simulink model "Car_14DOF_Lat_Long_Control_FINAL"  (R2024b)
settings: Solver=ode4  StartTime=0.0  StopTime=60  FixedStep=0.001  RelTol=1e-3
undefined symbols (not defined in the file): Ar1, Ar2, Ar3, Ar4, b, c, C_alpha, C_line, C_sigma, curvature, f, g, gradbp, Iw, Ix, Iy, Iz, k, ki, kp, kR, Kz1, Kz2, Kz3, L, L1, L2, lf, lh, lh_vis, lr, lw, m, mR, psi0, reff, uFz, Vx_ref, wc, x0, xRef2s, y0, yRef2s, z0
libraries: vehdynlibviscommon x1, deeplib x1
settings Model: Creator=sherlock2204  LastModifiedBy=sherlock2204
settings DebuggingCC: SigSpecEnsureSampleTimeMsg=none

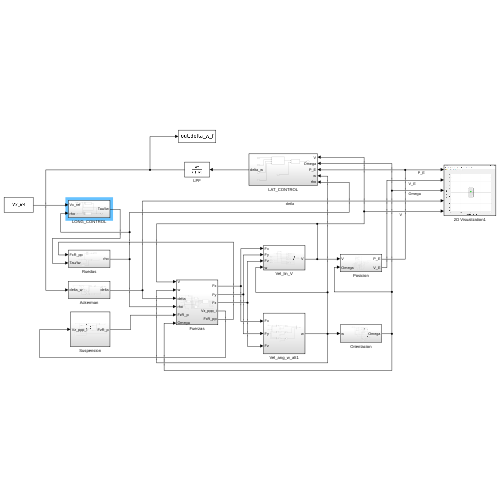
[thumbnail: Simulink's stored preview of the top-level diagram]
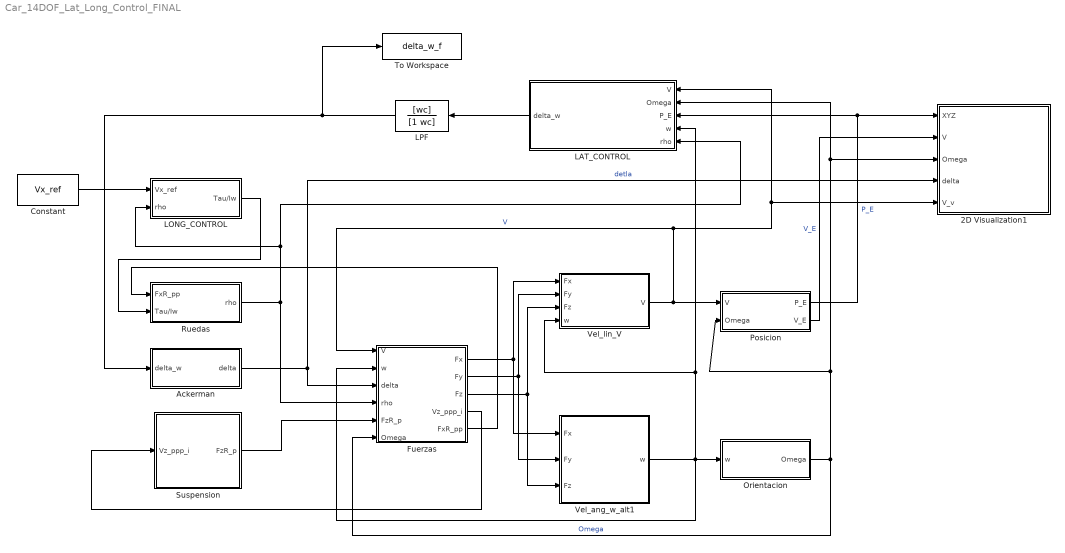
== system Car_14DOF_Lat_Long_Control_FINAL ==
  2D Visualization1 : Subsystem
      mask Display: image("visualization.JPG");
  Ackerman : Subsystem
  Constant : Constant  Value=Vx_ref
  Fuerzas : Subsystem
  LAT_CONTROL : Subsystem
  LONG_CONTROL : Subsystem
  LPF : TransferFcn  Numerator=[wc]  Denominator=[1 wc]
  Orientacion : Subsystem
  Posicion : Subsystem
  Ruedas : Subsystem
  Suspension : Subsystem
  To Workspace : ToWorkspace  VariableName=delta_w_f  SaveFormat=Timeseries  SampleTime=-1
  Vel_ang_w_alt1 : Subsystem
  Vel_lin_V : Subsystem
  wires:
  Fuerzas/3(Fz) -> Vel_ang_w_alt1/3(Fz), Vel_lin_V/3(Fz)
  Vel_ang_w_alt1/1(w) -> Vel_lin_V/4(w), LAT_CONTROL/4(w), Orientacion/1(w), Fuerzas/2(w)
  Vel_lin_V/1(V) -> Fuerzas/1(V), LAT_CONTROL/1(V), 2D Visualization1/5(V_v), Posicion/1(V)  "V"
  Suspension/1(FzR_p) -> Fuerzas/5(FzR_p)
  Fuerzas/4(Vz_ppp_i) -> Suspension/1(Vz_ppp_i)
  Ackerman/1(delta) -> Fuerzas/3(delta), 2D Visualization1/4(delta)  "detla"
  Fuerzas/1(Fx) -> Vel_ang_w_alt1/1(Fx), Vel_lin_V/1(Fx)
  Fuerzas/2(Fy) -> Vel_ang_w_alt1/2(Fy), Vel_lin_V/2(Fy)
  Orientacion/1(Omega) -> LAT_CONTROL/2(Omega), 2D Visualization1/3(Omega), Posicion/2(Omega), Fuerzas/6(Omega)  "Omega"
  Posicion/2(V_E) -> 2D Visualization1/2(V)  "V_E"
  Posicion/1(P_E) -> 2D Visualization1/1(XYZ), LAT_CONTROL/3(P_E)  "P_E"
  Fuerzas/5(FxR_pp) -> Ruedas/1(FxR_pp)
  Ruedas/1(rho) -> Fuerzas/4(rho), LAT_CONTROL/5(rho), LONG_CONTROL/2(rho)
  Constant/1 -> LONG_CONTROL/1(Vx_ref)
  LONG_CONTROL/1(Tau/Iw) -> Ruedas/2(Tau/Iw)
  LPF/1 -> To Workspace/1, Ackerman/1(delta_w)
  LAT_CONTROL/1(delta_w) -> LPF/1

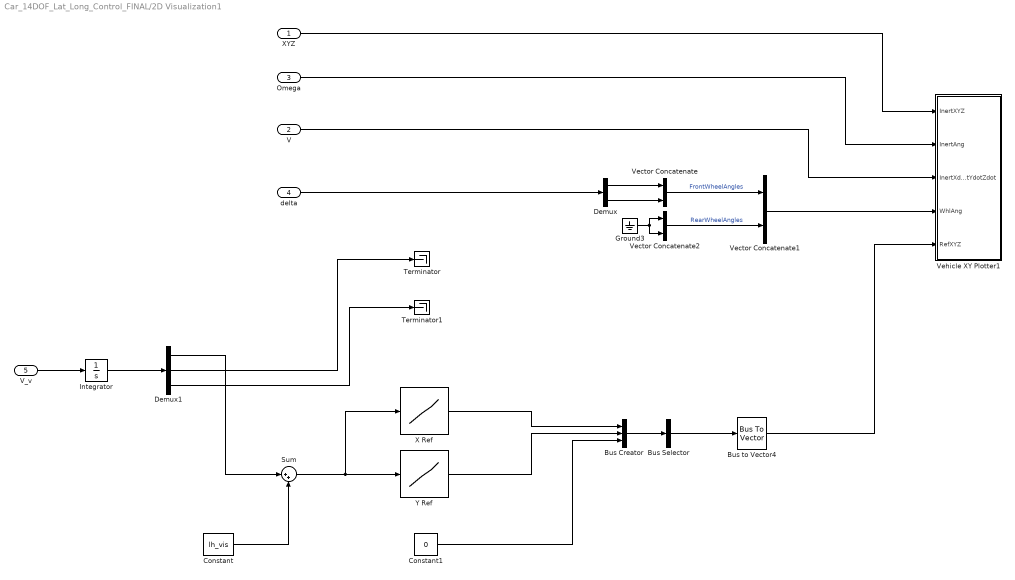
== system Car_14DOF_Lat_Long_Control_FINAL/2D Visualization1 ==
  XYZ : Inport
  V : Inport  Port=2
  Omega : Inport  Port=3
  delta : Inport  Port=4
  V_v : Inport  Port=5
  Bus Creator : BusCreator  Inputs=3
  Bus Selector : BusSelector  OutputSignals=signal1,signal2,signal3  OutputAsBus=on
  Bus to Vector4 : BusToVector
  Constant : Constant  Value=lh_vis
  Constant1 : Constant  Value=0
  Demux : Demux  Outputs=2
  Demux1 : Demux  Outputs=3
  Ground3 : Ground
  Integrator : Integrator
  Sum : Sum  Inputs=|++
  Terminator : Terminator
  Terminator1 : Terminator
  Vector Concatenate : Concatenate
  Vector Concatenate1 : Concatenate
  Vector Concatenate2 : Concatenate
  Vehicle XY Plotter1 : Subsystem  mask(Vehicle XY Plotter){extRef=on, extStats=off, extTireF=off, a=lf, b=lr, w=c, figBorder=10, bufferSize=1024, velNorm=5, tireFNorm=1000, pltDT=0.2}
      mask prompts: extRef "Plot path reference, extRef"; extStats "Display speed, RPM and Gear"; extTireF "Display tire forces"; a "Distance to front axle from CG, a [m]:"; b "Distance to rear axle from CG, b [m]:"; w "Track width, w [m]:"; figBorder "Distance to figure borders, figBorder [m]:"; bufferSize "Path buffer sampe size, bufferSize []:"; velNorm "Velocity vector scaling, velNorm [m*s/m]:"; tireFNorm "Tire force vector scaling, tireFNorm [m/N]:"; pltDT "Plot update rate, pltDT [s]:"
      mask help:
      | This block will display a MATLAB figure which indicates the vehicle path, current position and heading velocity.
      | An optional path reference is also provided.
      mask init:
      | block = gcb;
      | if autoblkschecksimstopped(block)
      |     ParamNames = {'extRef';'extStats';'extTireF';'extTireF'};
      |     PortNames = {'RefXYZ';'Stats';'TireFx';'TireFy'};
      |     for idx=1:length(PortNames)
      |         InportOption  = {'built-in/Ground', [PortNames{idx}, ' Ground'];...
      |             'built-in/Inport',PortNames{idx}};
      |         if ~strcmp(get_param(block,ParamNames{idx}),'on')
      |             NewBlkHdl = autoblksreplaceblock(block, InportOption, 1);
      |             set_param(NewBlkHdl, 'ShowName', 'off');
      |         else
      |             autoblksreplaceblock(block, InportOption, 2);
      |         end
      |     end
      |     InportNames = {'InertXYZ';'InertAng';'InertXdotYdotZdot';'WhlAng';'RefXYZ';'Stats';'TireFx';'TireFy'};
      |     FoundNames = get_param(find_system(block, 'LookUnderMasks', 'all', 'SearchDepth', 1, 'FollowLinks', 'on', 'BlockType', 'Inport'), 'Name');
      |     [~,PortI] = intersect(InportNames, FoundNames);
      |     PortI = sort(PortI);
      |     for idx = 1:length(PortI)
      |         set_param([block, '/', InportNames{PortI(idx)}], 'Port', num2str(idx));
      |     end
      | end
      mask TypeOptions a: Vehicle XY Plotter/a
      mask TypeOptions b: Vehicle XY Plotter/b
      mask TypeOptions w: Vehicle XY Plotter/w
      mask TypeOptions figBorder: Vehicle XY Plotter/figBorder
      mask TypeOptions bufferSize: Vehicle XY Plotter/bufferSize
      mask TypeOptions velNorm: Vehicle XY Plotter/velNorm
      mask TypeOptions tireFNorm: Vehicle XY Plotter/tireFNorm
      mask DialogControl Container3 Prompt: Plot and Display Options
  X Ref : Lookup_n-D  NumberOfTableDimensions=1  BreakpointsForDimension1=gradbp  Table=xRef2s  InternalRulePriority=Speed  RndMeth=Simplest
  Y Ref : Lookup_n-D  NumberOfTableDimensions=1  BreakpointsForDimension1=gradbp  Table=yRef2s  InternalRulePriority=Speed  RndMeth=Simplest
  wires:
  Omega/1 -> Vehicle XY Plotter1/2(InertAng)
  XYZ/1 -> Vehicle XY Plotter1/1(InertXYZ)
  V/1 -> Vehicle XY Plotter1/3(InertXdotYdotZdot)
  Vector Concatenate2/1 -> Vector Concatenate1/2  "RearWheelAngles"
  Vector Concatenate/1 -> Vector Concatenate1/1  "FrontWheelAngles"
  Ground3/1 -> Vector Concatenate2/2, Vector Concatenate2/1
  Vector Concatenate1/1 -> Vehicle XY Plotter1/4(WhlAng)
  delta/1 -> Demux/1
  Demux/1 -> Vector Concatenate/1
  Demux/2 -> Vector Concatenate/2
  Bus Creator/1 -> Bus Selector/1
  Y Ref/1 -> Bus Creator/2
  Bus Selector/1 -> Bus to Vector4/1
  Demux1/3 -> Terminator1/1
  X Ref/1 -> Bus Creator/1
  Constant1/1 -> Bus Creator/3
  Bus to Vector4/1 -> Vehicle XY Plotter1/5(RefXYZ)
  Demux1/2 -> Terminator/1
  V_v/1 -> Integrator/1
  Integrator/1 -> Demux1/1
  Demux1/1 -> Sum/1
  Sum/1 -> X Ref/1, Y Ref/1
  Constant/1 -> Sum/2

== system Car_14DOF_Lat_Long_Control_FINAL/Ackerman ==
  delta_w : Inport
  Atan : Trigonometry  Operator=atan
  Atan1 : Trigonometry  Operator=atan
  Constant : Constant  Value=L
  Divide : Product  Inputs=*/
  Divide1 : Product  Inputs=*/
  Gain : Gain  Gain=L
  Gain1 : Gain  Gain=lw
  Mux : Mux  Inputs=2
  Sum : Sum  Inputs=++|
  Sum1 : Sum  Inputs=-+|
  Tan : Trigonometry  Operator=tan
  delta : Outport
  wires:
  Mux/1 -> delta/1
  delta_w/1 -> Tan/1
  Tan/1 -> Gain/1, Gain1/1
  Gain/1 -> Divide1/1, Divide/1
  Divide/1 -> Atan/1
  Constant/1 -> Sum/2, Sum1/2
  Gain1/1 -> Sum/1, Sum1/1
  Sum/1 -> Divide/2
  Sum1/1 -> Divide1/2
  Divide1/1 -> Atan1/1
  Atan/1 -> Mux/1
  Atan1/1 -> Mux/2

== system Car_14DOF_Lat_Long_Control_FINAL/Fuerzas ==
  V : Inport
  w : Inport  Port=2
  delta : Inport  Port=3
  rho : Inport  Port=4
  FzR_p : Inport  Port=5
  Omega : Inport  Port=6
  Demux : Demux  Outputs=2
  Demux1 : Demux  Outputs=3
  M_Fuerzas : Subsystem
  Terminator : Terminator
  Vel_transf : Subsystem
  alpha_alt3 : Subsystem
  sigma_alt0 : Subsystem
  Fx : Outport
  Fy : Outport  Port=2
  Fz : Outport  Port=3
  Vz_ppp_i : Outport  Port=4
  FxR_pp : Outport  Port=5
  wires:
  V/1 -> Vel_transf/1(V)
  w/1 -> Vel_transf/2(w)
  Demux1/1 -> Vel_transf/3(phi), M_Fuerzas/5(phi)  "phi"
  Demux1/2 -> M_Fuerzas/6(theta), Vel_transf/4(theta)  "theta"
  M_Fuerzas/2(Fy) -> Fy/1
  M_Fuerzas/3(Fz) -> Fz/1
  delta/1 -> Vel_transf/5(delta), Demux/1
  Demux/2 -> alpha_alt3/4(delta_3), M_Fuerzas/4(delta_3)
  Demux/1 -> M_Fuerzas/3(delta_1), alpha_alt3/3(delta_1)
  rho/1 -> sigma_alt0/2(rho)
  Vel_transf/1(Vx_ppp_i) -> sigma_alt0/1(Vx_ppp_i)
  sigma_alt0/1(sigma) -> M_Fuerzas/1(sigma)
  alpha_alt3/1(alpha) -> M_Fuerzas/2(alpha)
  FzR_p/1 -> M_Fuerzas/7(FzR_p)
  Vel_transf/2(Vz_ppp_i) -> Vz_ppp_i/1
  Vel_transf/3(Vx_pp_i) -> alpha_alt3/1(Vx_pp_i)
  Vel_transf/4(Vy_pp_i) -> alpha_alt3/2(Vy_pp_i)
  Omega/1 -> Demux1/1
  Demux1/3 -> Terminator/1  "psi"
  M_Fuerzas/4(FxR_pp) -> FxR_pp/1
  M_Fuerzas/1(Fx) -> Fx/1

== system Car_14DOF_Lat_Long_Control_FINAL/LAT_CONTROL ==
  V : Inport
  Omega : Inport  Port=2
  P_E : Inport  Port=3
  w : Inport  Port=4
  rho : Inport  Port=5
  BACK_STEPPING_1 : Subsystem
  LSTM_NETWORK : Subsystem
  delta_w : Outport
  wires:
  V/1 -> BACK_STEPPING_1/1(V)
  Omega/1 -> BACK_STEPPING_1/2(Omega)
  P_E/1 -> BACK_STEPPING_1/3(P_E)
  w/1 -> BACK_STEPPING_1/4(w)
  rho/1 -> LSTM_NETWORK/2(rho)
  LSTM_NETWORK/1(delta_w) -> delta_w/1
  BACK_STEPPING_1/1(Tau_z) -> LSTM_NETWORK/1(Tau_z)

== system Car_14DOF_Lat_Long_Control_FINAL/LONG_CONTROL ==
  Vx_ref : Inport
  rho : Inport  Port=2
  ADRC : Subsystem
  ESO : Subsystem
  Tau/Iw : Outport
  wires:
  rho/1 -> ESO/1(x1), ADRC/1(x1)
  ADRC/1(u) -> Tau/Iw/1, ESO/2(u)  "u=Tau/Iw"
  ESO/1(hat_x2) -> ADRC/3(hat_x2)
  Vx_ref/1 -> ADRC/2(x1_ref)

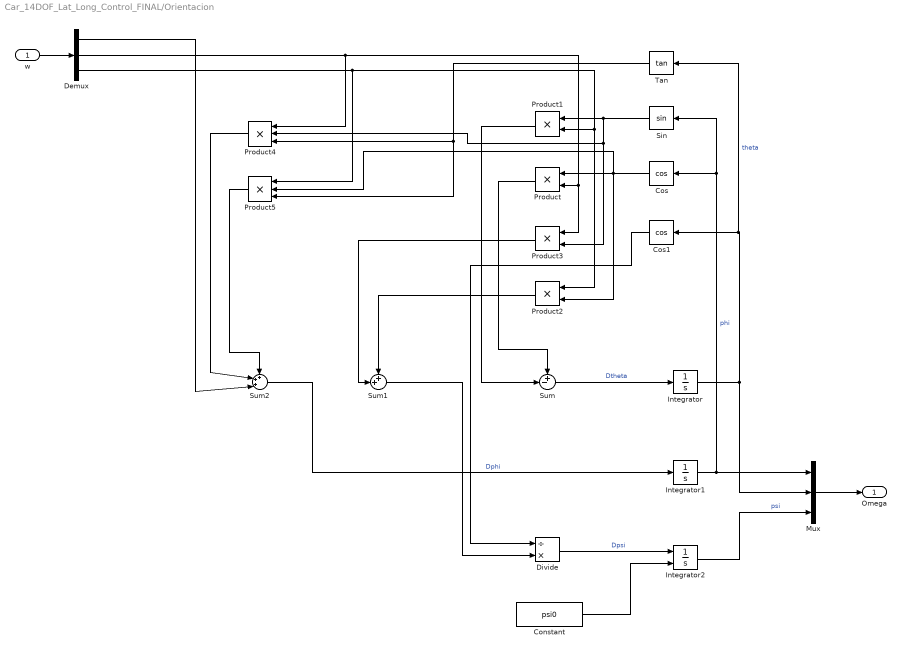
== system Car_14DOF_Lat_Long_Control_FINAL/Orientacion ==
  w : Inport
  Constant : Constant  Value=psi0
  Cos : Trigonometry  Operator=cos
  Cos1 : Trigonometry  Operator=cos
  Demux : Demux  Outputs=3
  Divide : Product  Inputs=/*
  Integrator : Integrator
  Integrator1 : Integrator
  Integrator2 : Integrator  InitialConditionSource=external
  Mux : Mux  Inputs=3
  Product{,1..3} (4 alike) : Product
  Product4 : Product  Inputs=3
  Product5 : Product  Inputs=3
  Sin : Trigonometry
  Sum : Sum  Inputs=+-|
  Sum1 : Sum  Inputs=++|
  Sum2 : Sum  Inputs=+++|
  Tan : Trigonometry  Operator=tan
  Omega : Outport
  wires:
  w/1 -> Demux/1
  Integrator/1 -> Mux/2, Tan/1, Cos1/1  "theta"
  Integrator2/1 -> Mux/3  "psi"
  Sin/1 -> Product4/2, Product3/2, Product1/1
  Cos/1 -> Product5/2, Product2/2, Product/1
  Demux/2 -> Product4/1, Product3/1, Product/2
  Demux/3 -> Product5/1, Product2/1, Product1/2
  Product/1 -> Sum/1
  Product1/1 -> Sum/2
  Sum/1 -> Integrator/1  "Dtheta"
  Integrator1/1 -> Sin/1, Cos/1, Mux/1  "phi"
  Product2/1 -> Sum1/1
  Product3/1 -> Sum1/2
  Divide/1 -> Integrator2/1  "Dpsi"
  Sum1/1 -> Divide/2
  Cos1/1 -> Divide/1
  Tan/1 -> Product4/3, Product5/3
  Sum2/1 -> Integrator1/1  "Dphi"
  Product5/1 -> Sum2/1
  Product4/1 -> Sum2/2
  Demux/1 -> Sum2/3
  Mux/1 -> Omega/1
  Constant/1 -> Integrator2/2

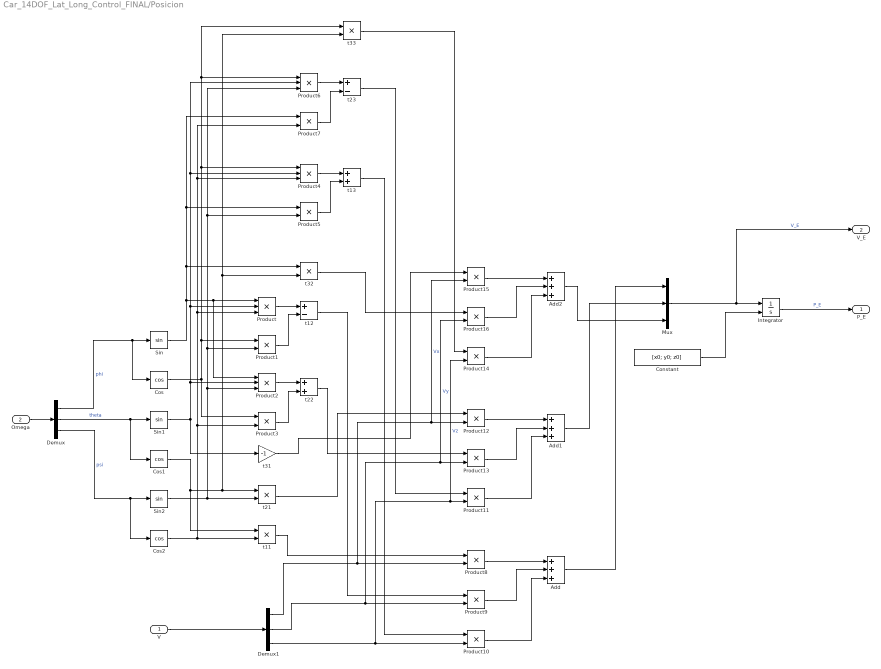
== system Car_14DOF_Lat_Long_Control_FINAL/Posicion ==
  V : Inport
  Omega : Inport  Port=2
  Add : Sum  Inputs=+++
  Add1 : Sum  Inputs=+++
  Add2 : Sum  Inputs=+++
  Constant : Constant  Value=[x0; y0; z0]
  Cos : Trigonometry  Operator=cos
  Cos1 : Trigonometry  Operator=cos
  Cos2 : Trigonometry  Operator=cos
  Demux : Demux  Outputs=3
  Demux1 : Demux  Outputs=3
  Integrator : Integrator  InitialConditionSource=external
  Mux : Mux  Inputs=3
  Product{,2,4,6} (4 alike) : Product  Inputs=3
  Product{1,3,5,7..16} (13 alike) : Product
  Sin : Trigonometry
  Sin1 : Trigonometry
  Sin2 : Trigonometry
  t{11,21,32..33} (4 alike) : Product
  t12 : Sum  Inputs=+-
  t13 : Sum
  t22 : Sum
  t23 : Sum  Inputs=+-
  t31 : Gain  Gain=-1
  P_E : Outport
  V_E : Outport  Port=2
  wires:
  Demux/1 -> Cos/1, Sin/1  "phi"
  Demux/2 -> Cos1/1, Sin1/1  "theta"
  Demux/3 -> Cos2/1, Sin2/1  "psi"
  Omega/1 -> Demux/1
  Cos2/1 -> Product7/2, Product4/3, Product/3, Product3/2, t11/2
  Cos1/1 -> t21/1, t33/2, t32/2, t11/1
  Sin2/1 -> Product6/3, Product5/2, Product1/2, Product2/3, t21/2
  Sin1/1 -> Product6/2, Product4/2, Product/2, Product2/2, t31/1
  Sin/1 -> Product7/1, Product5/1, t32/1, Product2/1, Product/1
  Cos/1 -> t33/1, Product6/1, Product4/1, Product1/1, Product3/1
  Product/1 -> t12/1
  Product1/1 -> t12/2
  Product3/1 -> t22/2
  Product2/1 -> t22/1
  Product5/1 -> t13/2
  Product4/1 -> t13/1
  Product6/1 -> t23/1
  Product7/1 -> t23/2
  V/1 -> Demux1/1
  Demux1/1 -> Product15/2, Product12/2, Product8/2  "Vx"
  Demux1/3 -> Product10/2, Product14/2, Product11/2  "Vz"
  Demux1/2 -> Product9/2, Product16/2, Product13/2  "Vy"
  t11/1 -> Product8/1
  t12/1 -> Product9/1
  t13/1 -> Product10/1
  Product8/1 -> Add/1
  Product9/1 -> Add/2
  Product10/1 -> Add/3
  Product13/1 -> Add1/2
  Product12/1 -> Add1/1
  Product11/1 -> Add1/3
  t21/1 -> Product12/1
  t22/1 -> Product13/1
  t23/1 -> Product11/1
  Product15/1 -> Add2/1
  Product16/1 -> Add2/2
  Product14/1 -> Add2/3
  t31/1 -> Product15/1
  t32/1 -> Product16/1
  t33/1 -> Product14/1
  Add/1 -> Mux/1
  Add1/1 -> Mux/2
  Add2/1 -> Mux/3
  Mux/1 -> V_E/1, Integrator/1  "V_E"
  Integrator/1 -> P_E/1  "P_E"
  Constant/1 -> Integrator/2

== system Car_14DOF_Lat_Long_Control_FINAL/Ruedas ==
  FxR_pp : Inport
  Tau/Iw : Inport  Port=2
  Add1 : Sum  Inputs=++++
  Constant : Constant  Value=0.0001*[1 1 1 1]
  Demux : Demux
  Gain : Gain
  Gain13 : Gain  Gain=reff/Iw
  Gain3 : Gain  Gain=1/4
  Integrator4 : Integrator  InitialConditionSource=external
  Sum : Sum  Inputs=|+-
  To Workspace : ToWorkspace  VariableName=tau_w  SaveFormat=Timeseries  SampleTime=-1
  rho : Outport
  wires:
  FxR_pp/1 -> Gain13/1
  Tau/Iw/1 -> Gain/1  "u=Tau/Iw"
  Sum/1 -> Integrator4/1  "Drho"
  Gain13/1 -> Sum/2  "EPS(t)"
  Gain/1 -> Demux/1, Sum/1  "Tau"
  Integrator4/1 -> rho/1
  Constant/1 -> Integrator4/2
  Add1/1 -> Gain3/1
  Demux/3 -> Add1/3
  Demux/2 -> Add1/2
  Demux/1 -> Add1/1
  Demux/4 -> Add1/4
  Gain3/1 -> To Workspace/1

== system Car_14DOF_Lat_Long_Control_FINAL/Suspension ==
  Vz_ppp_i : Inport
  Add : Sum  Inputs=--
  Add1 : Sum  Inputs=++-
  Constant2 : Constant  Value=[0;0;0;0]
  Constant3 : Constant  Value=[0;0;0;0]
  Constant4 : Constant  Value=[0;0;0;0]
  Gain : Gain  Gain=b
  Gain1 : Gain  Gain=k
  Gain4 : Gain  Gain=1/mR
  Gain7 : Gain  Gain=kR
  Integrator2 : Integrator  InitialConditionSource=external
  Integrator3 : Integrator  InitialConditionSource=external
  Integrator4 : Integrator  InitialConditionSource=external
  Sum : Sum  Inputs=|+-
  Sum2 : Sum  Inputs=|+-
  FzR_p : Outport
  wires:
  Sum/1 -> Gain/1
  Integrator3/1 -> Gain7/1, Sum2/2  "zR"
  Sum2/1 -> Gain1/1
  Add/1 -> FzR_p/1
  Add1/1 -> Gain4/1
  Gain/1 -> Add1/1, Add/1
  Integrator2/1 -> Integrator3/1, Sum/2  "DzR"
  Gain1/1 -> Add1/2, Add/2
  Gain4/1 -> Integrator2/1
  Constant4/1 -> Integrator2/2
  Constant3/1 -> Integrator3/2
  Vz_ppp_i/1 -> Integrator4/1, Sum/1  "DzA"
  Integrator4/1 -> Sum2/1  "zA"
  Constant2/1 -> Integrator4/2
  Gain7/1 -> Add1/3

== system Car_14DOF_Lat_Long_Control_FINAL/Vel_ang_w_alt1 ==
  Fx : Inport
  Fy : Inport  Port=2
  Fz : Inport  Port=3
  Integrator : Integrator  InitialConditionSource=external
  Integrator1 : Integrator  InitialConditionSource=external
  Integrator2 : Integrator  InitialConditionSource=external
  Multiply : Gain  Gain=(1/Ix)*[c c -c -c lh lh lh lh]  Multiplication=Matrix(K*u) (u vector)
  Multiply1 : Gain  Gain=(1/Iy)*[-lh -lh -lh -lh -lf lr -lf lr]  Multiplication=Matrix(K*u) (u vector)
  Multiply2 : Gain  Gain=(1/Iz)*[lf -lr lf -lr -c -c c c]  Multiplication=Matrix(K*u) (u vector)
  Mux : Mux  Inputs=3
  Vector Concatenate : Concatenate
  Vector Concatenate1 : Concatenate
  Vector Concatenate2 : Concatenate
  wx0 : Constant  Value=0
  wy0 : Constant  Value=0
  wz0 : Constant  Value=0
  w : Outport
  wires:
  wx0/1 -> Integrator/2
  wy0/1 -> Integrator1/2
  Mux/1 -> w/1
  wz0/1 -> Integrator2/2
  Integrator/1 -> Mux/1  "wx"
  Fz/1 -> Vector Concatenate/1, Vector Concatenate1/2
  Fy/1 -> Vector Concatenate/2, Vector Concatenate2/1
  Vector Concatenate/1 -> Multiply/1
  Multiply1/1 -> Integrator1/1
  Vector Concatenate1/1 -> Multiply1/1
  Fx/1 -> Vector Concatenate2/2, Vector Concatenate1/1
  Integrator1/1 -> Mux/2  "wy"
  Vector Concatenate2/1 -> Multiply2/1
  Integrator2/1 -> Mux/3  "wz"
  Multiply/1 -> Integrator/1
  Multiply2/1 -> Integrator2/1

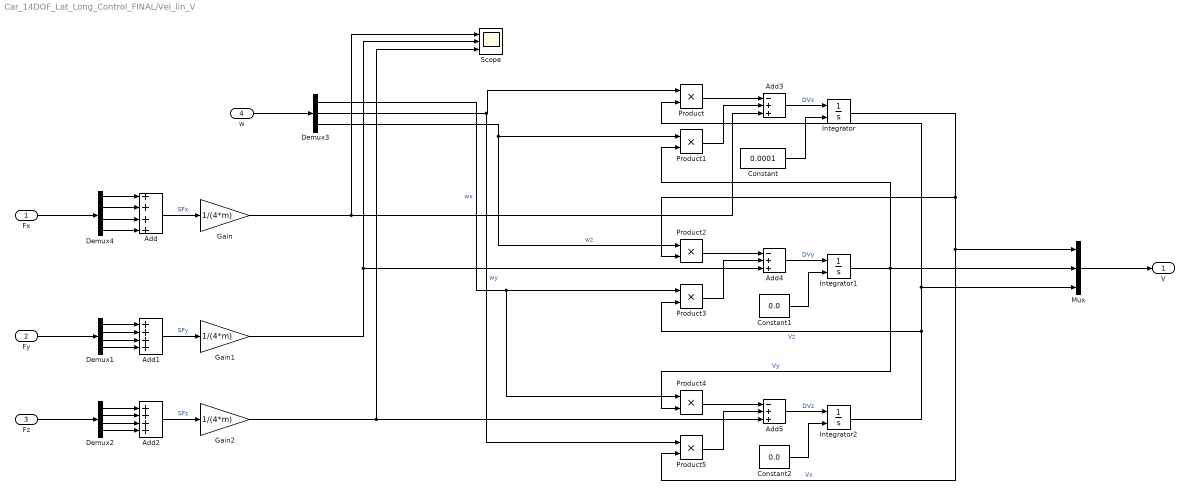
== system Car_14DOF_Lat_Long_Control_FINAL/Vel_lin_V ==
  Fx : Inport
  Fy : Inport  Port=2
  Fz : Inport  Port=3
  w : Inport  Port=4
  Add : Sum  Inputs=++++
  Add1 : Sum  Inputs=++++
  Add2 : Sum  Inputs=++++
  Add3 : Sum  Inputs=-++
  Add4 : Sum  Inputs=-++
  Add5 : Sum  Inputs=-++
  Constant : Constant  Value=0.0001  SampleTime=0.001
  Constant1 : Constant  Value=0.0
  Constant2 : Constant  Value=0.0
  Demux1 : Demux
  Demux2 : Demux
  Demux3 : Demux  Outputs=3
  Demux4 : Demux
  Gain : Gain  Gain=1/(4*m)
  Gain1 : Gain  Gain=1/(4*m)
  Gain2 : Gain  Gain=1/(4*m)
  Integrator : Integrator  InitialConditionSource=external  UpperSaturationLimit=27.7778  LowerSaturationLimit=-27.7778  AbsoluteTolerance=10
  Integrator1 : Integrator  InitialConditionSource=external
  Integrator2 : Integrator  InitialConditionSource=external
  Mux : Mux  Inputs=3
  Product{,1..5} (6 alike) : Product
  Scope : Scope  NumInputPorts=3
  V : Outport
  wires:
  Fy/1 -> Demux1/1
  Demux1/1 -> Add1/1
  Demux1/2 -> Add1/2
  Demux1/3 -> Add1/3
  Demux1/4 -> Add1/4
  Demux2/1 -> Add2/1
  Fz/1 -> Demux2/1
  Demux2/2 -> Add2/2
  Demux2/4 -> Add2/4
  Demux2/3 -> Add2/3
  w/1 -> Demux3/1
  Add/1 -> Gain/1  "SFx"
  Add1/1 -> Gain1/1  "SFy"
  Add2/1 -> Gain2/1  "SFz"
  Add3/1 -> Integrator/1  "DVx"
  Product1/1 -> Add3/2
  Product/1 -> Add3/1
  Demux3/3 -> Product2/1, Product1/1  "wz"
  Demux3/2 -> Product5/1, Product/1  "wy"
  Product2/1 -> Add4/1
  Add4/1 -> Integrator1/1  "DVy"
  Product3/1 -> Add4/2
  Add5/1 -> Integrator2/1  "DVz"
  Product4/1 -> Add5/1
  Product5/1 -> Add5/2
  Demux3/1 -> Product4/1, Product3/1  "wx"
  Integrator1/1 -> Mux/2, Product1/2, Product4/2  "Vy"
  Integrator2/1 -> Product3/2, Mux/3, Product/2  "Vz"
  Integrator/1 -> Mux/1, Product5/2, Product2/2  "Vx"
  Mux/1 -> V/1
  Demux4/1 -> Add/1
  Demux4/4 -> Add/4
  Demux4/2 -> Add/2
  Demux4/3 -> Add/3
  Fx/1 -> Demux4/1
  Constant/1 -> Integrator/2
  Constant1/1 -> Integrator1/2
  Constant2/1 -> Integrator2/2
  Gain/1 -> Scope/1, Add3/3
  Gain1/1 -> Scope/2, Add4/3
  Gain2/1 -> Scope/3, Add5/3

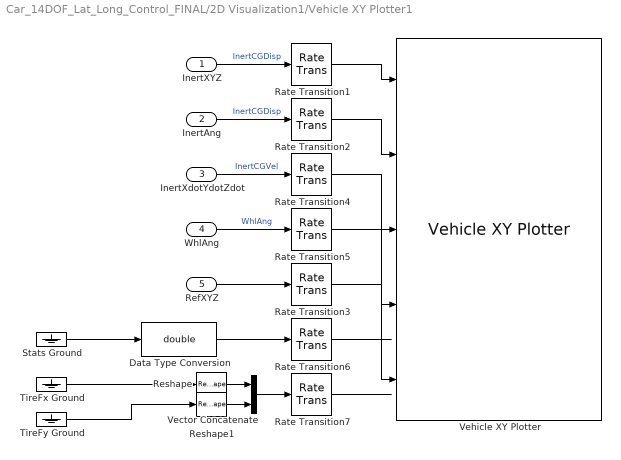
== system Car_14DOF_Lat_Long_Control_FINAL/2D Visualization1/Vehicle XY Plotter1 ==
  InertXYZ : Inport
  InertAng : Inport  Port=2
  InertXdotYdotZdot : Inport  Port=3
  WhlAng : Inport  Port=4
  RefXYZ : Inport  Port=5
  Data Type Conversion : DataTypeConversion  OutDataTypeStr=double  SaturateOnIntegerOverflow=off  RndMeth=Floor
  Rate Transition{1..7} (7 alike) : RateTransition  Deterministic=off  OutPortSampleTime=pltDT
  Reshape : Reshape  OutputDimensionality=Row vector (2-D)
  Reshape1 : Reshape  OutputDimensionality=Row vector (2-D)
  Stats Ground : Ground
  TireFx Ground : Ground
  TireFy Ground : Ground
  Vector Concatenate : Concatenate  Mode=Multidimensional array
  Vehicle XY Plotter : vehdynlibviscommon/Vehicle XY Plotter  w=w  a=a  b=b  figBorder=figBorder  bufferSize=bufferSize  extStats=off  extTireF=off
  wires:
  Stats Ground/1 -> Data Type Conversion/1
  InertAng/1 -> Rate Transition2/1  "InertCGDisp"
  InertXdotYdotZdot/1 -> Rate Transition4/1  "InertCGVel"
  InertXYZ/1 -> Rate Transition1/1  "InertCGDisp"
  WhlAng/1 -> Rate Transition5/1  "WhlAng"
  Rate Transition3/1 -> Vehicle XY Plotter/5
  Rate Transition1/1 -> Vehicle XY Plotter/1
  Rate Transition2/1 -> Vehicle XY Plotter/2
  Rate Transition4/1 -> Vehicle XY Plotter/3
  Rate Transition5/1 -> Vehicle XY Plotter/4
  Rate Transition6/1 -> ?
  Data Type Conversion/1 -> Rate Transition6/1
  Rate Transition7/1 -> ?
  Reshape/1 -> Vector Concatenate/1
  Reshape1/1 -> Vector Concatenate/2
  Vector Concatenate/1 -> Rate Transition7/1
  TireFx Ground/1 -> Reshape/1
  TireFy Ground/1 -> Reshape1/1
  RefXYZ/1 -> Rate Transition3/1

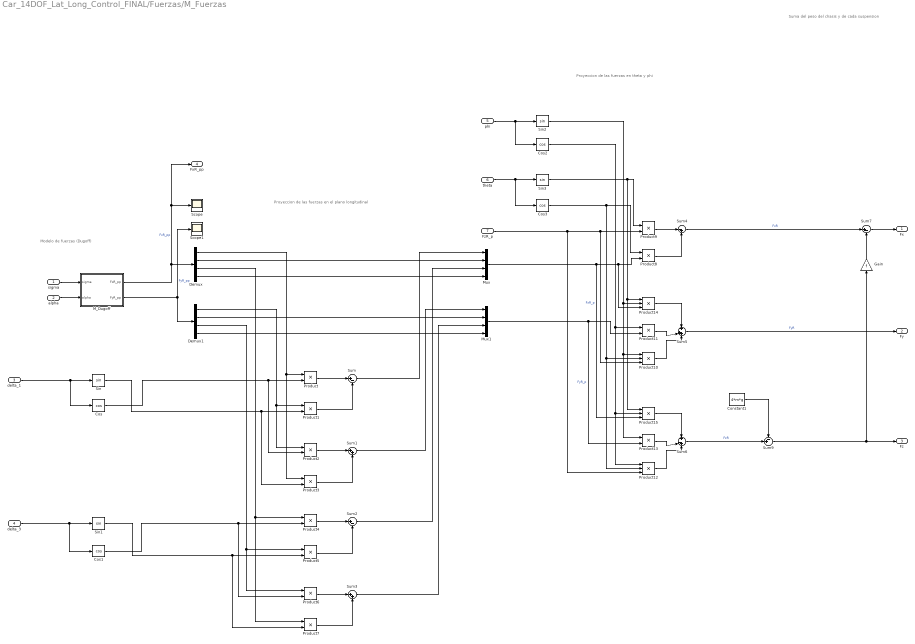
== system Car_14DOF_Lat_Long_Control_FINAL/Fuerzas/M_Fuerzas ==
  note: Modelo de fuerzas (Dugoff)
  note: Suma del peso del chasis
      | y de cada suspension
  note: Proyeccion de las fuerzas en theta y phi
  note: Proyeccion de las fuerzas en el plano longitudinal
  sigma : Inport
  alpha : Inport  Port=2
  delta_1 : Inport  Port=3
  delta_3 : Inport  Port=4
  phi : Inport  Port=5
  theta : Inport  Port=6
  FzR_p : Inport  Port=7
  Constant1 : Constant  Value=4*m*g
  Cos{,1..3} (4 alike) : Trigonometry  Operator=cos
  Demux : Demux
  Demux1 : Demux
  Gain : Gain  Gain=f
  M_Dugoff : Subsystem
  Mux : Mux
  Mux1 : Mux
  Product{,1..9,11,13} (12 alike) : Product
  Product{10,12,14..15} (4 alike) : Product  Inputs=3
  Scope : Scope
  Scope1 : Scope
  Sin{,1..3} (4 alike) : Trigonometry
  Sum : Sum  Inputs=|+-
  Sum1 : Sum  Inputs=|++
  Sum2 : Sum  Inputs=|+-
  Sum3 : Sum  Inputs=|++
  Sum4 : Sum  Inputs=|-+
  Sum5 : Sum  Inputs=+|++
  Sum6 : Sum  Inputs=+|-+
  Sum7 : Sum  Inputs=|+-
  Sum9 : Sum  Inputs=-+|
  Fx : Outport
  Fy : Outport  Port=2
  Fz : Outport  Port=3
  FxR_pp : Outport  Port=4
  wires:
  M_Dugoff/2(FyR_pp) -> Demux1/1, Scope1/1  "FyR_pp"
  Demux/2 -> Mux/2
  Demux/4 -> Mux/4
  Demux1/2 -> Mux1/2
  Demux1/4 -> Mux1/4
  Demux/1 -> Product3/1, Product/1
  Cos/1 -> Product2/2, Product/2
  Product/1 -> Sum/1
  Sin/1 -> Product3/2, Product1/2
  Demux1/1 -> Product2/1, Product1/1
  Product1/1 -> Sum/2
  Sum/1 -> Mux/1
  Product2/1 -> Sum1/1
  Product3/1 -> Sum1/2
  Sum1/1 -> Mux1/1
  Product6/1 -> Sum3/1
  Product7/1 -> Sum3/2
  Product5/1 -> Sum2/2
  Product4/1 -> Sum2/1
  Demux/3 -> Product7/1, Product4/1
  Demux1/3 -> Product6/1, Product5/1
  Cos1/1 -> Product6/2, Product4/2
  Sin1/1 -> Product7/2, Product5/2
  Sum2/1 -> Mux/3
  Sum3/1 -> Mux1/3
  Mux/1 -> Product15/3, Product14/3, Product8/2  "FxR_p"
  FzR_p/1 -> Product12/3, Product9/2, Product10/3
  Cos3/1 -> Product12/2, Product10/2, Product8/1
  Sin3/1 -> Product15/1, Product14/1, Product9/1
  Product9/1 -> Sum4/1
  Product8/1 -> Sum4/2
  Product10/1 -> Sum5/3
  Sum5/1 -> Fy/1  "FyR"
  Product11/1 -> Sum5/2
  Product13/1 -> Sum6/2
  Product12/1 -> Sum6/3
  Sum6/1 -> Sum9/2  "FzR"
  Product14/1 -> Sum5/1
  Sin2/1 -> Product13/1, Product10/1, Product14/2
  Mux1/1 -> Product11/2, Product13/2  "FyR_p"
  Cos2/1 -> Product11/1, Product12/1, Product15/2
  Product15/1 -> Sum6/1
  Sum4/1 -> Sum7/1  "FxR"
  sigma/1 -> M_Dugoff/1(sigma)
  alpha/1 -> M_Dugoff/2(alpha)
  M_Dugoff/1(FxR_pp) -> Scope/1, FxR_pp/1, Demux/1  "FxR_pp"
  Sum9/1 -> Gain/1, Fz/1
  phi/1 -> Cos2/1, Sin2/1
  theta/1 -> Cos3/1, Sin3/1
  delta_1/1 -> Cos/1, Sin/1
  delta_3/1 -> Cos1/1, Sin1/1
  Constant1/1 -> Sum9/1
  Sum7/1 -> Fx/1
  Gain/1 -> Sum7/2

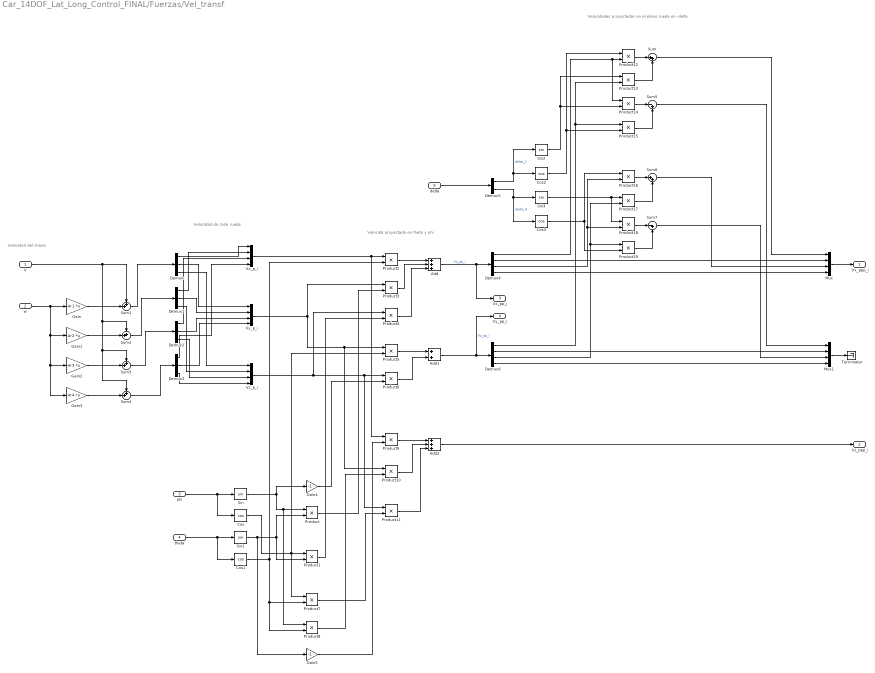
== system Car_14DOF_Lat_Long_Control_FINAL/Fuerzas/Vel_transf ==
  note: Velocidades proyectadas en el plano rueda en -delta
  note: Velocida proyectada en theta y phi
  note: Velocidad de cada rueda
  note: Velocidad del chasis
  V : Inport
  w : Inport  Port=2
  phi : Inport  Port=3
  theta : Inport  Port=4
  delta : Inport  Port=5
  Add : Sum  Inputs=+++
  Add1 : Sum
  Add2 : Sum  Inputs=+++
  Cos{,1..3} (4 alike) : Trigonometry  Operator=cos
  Demux{,1..3} (4 alike) : Demux  Outputs=3
  Demux4 : Demux
  Demux5 : Demux  Outputs=2
  Demux6 : Demux
  Gain : Gain  Gain=Ar1  Multiplication=Matrix(K*u)
  Gain1 : Gain  Gain=Ar2  Multiplication=Matrix(K*u)
  Gain2 : Gain  Gain=Ar3  Multiplication=Matrix(K*u)
  Gain3 : Gain  Gain=Ar4  Multiplication=Matrix(K*u)
  Gain4 : Gain  Gain=-1
  Gain5 : Gain  Gain=-1
  Mux : Mux
  Mux1 : Mux
  Product{,1..19} (20 alike) : Product
  Sin{,1..3} (4 alike) : Trigonometry
  Sum : Sum  Inputs=|++
  Sum{1..4} (4 alike) : Sum  Inputs=++|
  Sum5 : Sum  Inputs=|-+
  Sum6 : Sum  Inputs=|++
  Sum7 : Sum  Inputs=|-+
  Terminator : Terminator
  Vx_p_i : Mux
  Vy_p_i : Mux
  Vz_p_i : Mux
  Vx_ppp_i : Outport
  Vz_ppp_i : Outport  Port=2
  Vx_pp_i : Outport  Port=3
  Vy_pp_i : Outport  Port=4
  wires:
  w/1 -> Gain3/1, Gain2/1, Gain1/1, Gain/1
  Gain/1 -> Sum1/2
  Gain1/1 -> Sum2/2
  V/1 -> Sum2/1, Sum4/1, Sum3/1, Sum1/1
  Gain2/1 -> Sum3/2
  Gain3/1 -> Sum4/2
  Sum1/1 -> Demux/1
  Sum2/1 -> Demux1/1
  Sum3/1 -> Demux2/1
  Sum4/1 -> Demux3/1
  Demux/1 -> Vx_p_i/1
  Demux1/1 -> Vx_p_i/2
  Demux2/1 -> Vx_p_i/3
  Demux3/1 -> Vx_p_i/4
  Demux/2 -> Vy_p_i/1
  Demux1/2 -> Vy_p_i/2
  Demux2/2 -> Vy_p_i/3
  Demux3/2 -> Vy_p_i/4
  Demux/3 -> Vz_p_i/1
  Demux1/3 -> Vz_p_i/2
  Demux2/3 -> Vz_p_i/3
  Demux3/3 -> Vz_p_i/4
  Sin1/1 -> Gain5/1, Product1/2, Product/2
  Cos/1 -> Product7/1, Product1/1, Product5/2
  Sin/1 -> Gain4/1, Product8/1, Product/1
  Vx_p_i/1 -> Product9/1, Product2/1
  Cos1/1 -> Product8/2, Product7/2, Product2/2
  Product2/1 -> Add/1
  Product3/1 -> Add/2
  Product/1 -> Product3/2
  Vy_p_i/1 -> Product10/1, Product5/1, Product3/1
  Vz_p_i/1 -> Product4/1, Product11/1, Product6/1
  Product1/1 -> Product4/2
  Product4/1 -> Add/3
  Product5/1 -> Add1/1
  Gain4/1 -> Product6/2
  Product6/1 -> Add1/2
  Add2/1 -> Vz_ppp_i/1
  Product9/1 -> Add2/1
  Gain5/1 -> Product9/2
  Product10/1 -> Add2/2
  Product8/1 -> Product10/2
  Product11/1 -> Add2/3
  Product7/1 -> Product11/2
  Add/1 -> Vx_pp_i/1, Demux4/1  "Vx_pp_i"
  Add1/1 -> Vy_pp_i/1, Demux6/1  "Vy_pp_i"
  Mux/1 -> Vx_ppp_i/1
  Demux4/2 -> Mux/2
  Demux4/4 -> Mux/4
  Demux6/2 -> Mux1/2
  Demux6/4 -> Mux1/4
  Demux5/1 -> Cos2/1, Sin2/1  "delta_1"
  Demux5/2 -> Sin3/1, Cos3/1  "delta_3"
  Cos2/1 -> Product15/2, Product12/1
  Product12/1 -> Sum/1
  Product13/1 -> Sum/2
  Product14/1 -> Sum5/1
  Product15/1 -> Sum5/2
  Sin2/1 -> Product14/2, Product13/1
  Product16/1 -> Sum6/1
  Product17/1 -> Sum6/2
  Product19/1 -> Sum7/2
  Product18/1 -> Sum7/1
  Demux4/1 -> Product12/2, Product14/1
  Demux6/1 -> Product13/2, Product15/1
  Sum/1 -> Mux/1
  Sum5/1 -> Mux1/1
  Cos3/1 -> Product19/2, Product16/1
  Demux4/3 -> Product18/2, Product16/2
  Demux6/3 -> Product19/1, Product17/2
  Sin3/1 -> Product18/1, Product17/1
  Sum6/1 -> Mux/3
  Sum7/1 -> Mux1/3
  Mux1/1 -> Terminator/1
  phi/1 -> Cos/1, Sin/1
  theta/1 -> Cos1/1, Sin1/1
  delta/1 -> Demux5/1

== system Car_14DOF_Lat_Long_Control_FINAL/Fuerzas/alpha_alt3 ==
  Vx_pp_i : Inport
  Vy_pp_i : Inport  Port=2
  delta_1 : Inport  Port=3
  delta_3 : Inport  Port=4
  Atan{,1..3} (4 alike) : Trigonometry  Operator=atan
  Demux : Demux
  Demux1 : Demux
  Divide{,1..3} (4 alike) : Product  Inputs=*/
  Gain : Gain
  Gain1 : Gain
  Mux : Mux
  Sum1 : Sum  Inputs=-+|
  Sum2 : Sum  Inputs=-+|
  alpha : Outport
  wires:
  Vx_pp_i/1 -> Demux/1
  Vy_pp_i/1 -> Demux1/1
  Demux1/1 -> Divide/1
  Demux/1 -> Divide/2
  Divide/1 -> Atan/1
  delta_1/1 -> Sum2/1
  Sum2/1 -> Mux/1
  Divide1/1 -> Atan1/1
  Gain/1 -> Mux/2
  Demux1/2 -> Divide1/1
  Demux/2 -> Divide1/2
  Divide2/1 -> Atan3/1
  Divide3/1 -> Atan2/1
  Demux1/4 -> Divide2/1
  Demux/4 -> Divide2/2
  Gain1/1 -> Mux/4
  Sum1/1 -> Mux/3
  Demux1/3 -> Divide3/1
  Demux/3 -> Divide3/2
  delta_3/1 -> Sum1/1
  Atan/1 -> Sum2/2
  Atan1/1 -> Gain/1
  Atan2/1 -> Sum1/2
  Atan3/1 -> Gain1/1
  Mux/1 -> alpha/1

== system Car_14DOF_Lat_Long_Control_FINAL/Fuerzas/sigma_alt0 ==
  Vx_ppp_i : Inport
  rho : Inport  Port=2
  Add{,1..3} (4 alike) : Sum  Inputs=-+
  Demux : Demux
  Demux1 : Demux
  Divide{,1..3} (4 alike) : Product  Inputs=/*
  Gain : Gain  Gain=reff
  Max{,1..3} (4 alike) : MinMax  Function=max  Inputs=2
  Mux : Mux
  sigma : Outport
  wires:
  Add2/1 -> Divide/2
  Max/1 -> Divide/1
  Max1/1 -> Divide1/1
  Add1/1 -> Divide1/2
  Add/1 -> Divide2/2
  Max2/1 -> Divide2/1
  Gain/1 -> Demux/1
  Mux/1 -> sigma/1
  rho/1 -> Gain/1
  Vx_ppp_i/1 -> Demux1/1
  Demux/1 -> Max2/2, Add/2  "rho_1"
  Demux1/1 -> Max2/1, Add/1
  Divide2/1 -> Mux/1
  Divide1/1 -> Mux/2
  Demux/2 -> Max1/2, Add1/2  "rho_2"
  Demux1/2 -> Max1/1, Add1/1
  Divide/1 -> Mux/3
  Max3/1 -> Divide3/1
  Add3/1 -> Divide3/2
  Divide3/1 -> Mux/4
  Demux/3 -> Max/2, Add2/2  "rho_3"
  Demux1/3 -> Max/1, Add2/1
  Demux/4 -> Max3/2, Add3/2  "rho_4"
  Demux1/4 -> Max3/1, Add3/1  "rho_4"

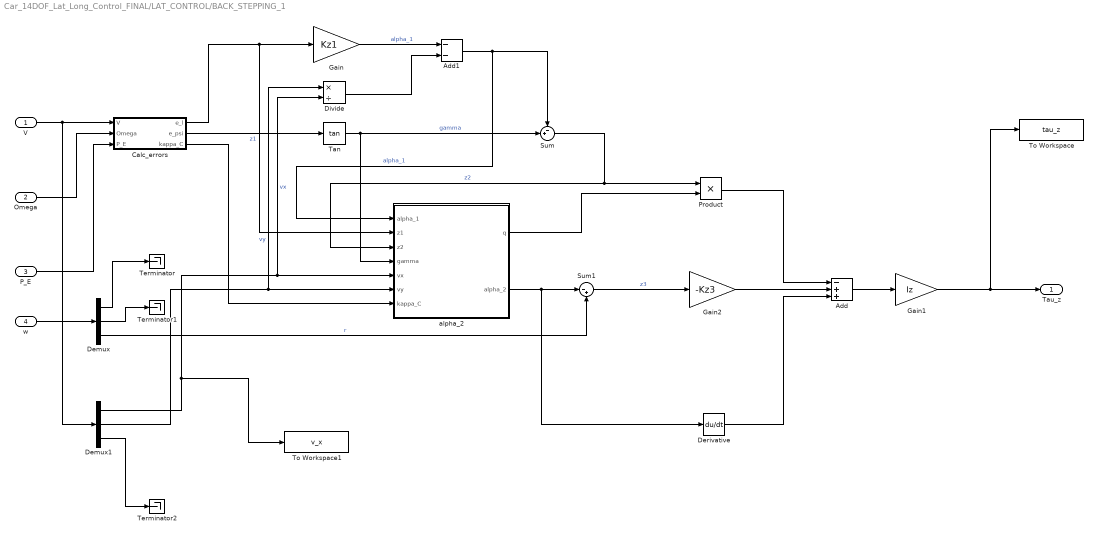
== system Car_14DOF_Lat_Long_Control_FINAL/LAT_CONTROL/BACK_STEPPING_1 ==
  V : Inport
  Omega : Inport  Port=2
  P_E : Inport  Port=3
  w : Inport  Port=4
  Add : Sum  Inputs=-++
  Add1 : Sum  Inputs=--
  Calc_errors : Subsystem
  Demux : Demux  Outputs=3
  Demux1 : Demux  Outputs=3
  Derivative : Derivative
  Divide : Product  Inputs=*/
  Gain : Gain  Gain=Kz1
  Gain1 : Gain  Gain=Iz
  Gain2 : Gain  Gain=-Kz3
  Product : Product
  Sum : Sum  Inputs=-+|
  Sum1 : Sum  Inputs=|-+
  Tan : Trigonometry  Operator=tan
  Terminator : Terminator
  Terminator1 : Terminator
  Terminator2 : Terminator
  To Workspace : ToWorkspace  VariableName=tau_z  SaveFormat=Timeseries  SampleTime=-1
  To Workspace1 : ToWorkspace  VariableName=v_x  SaveFormat=Timeseries  SampleTime=-1
  alpha_2 : Subsystem
  Tau_z : Outport
  wires:
  V/1 -> Calc_errors/1(V), Demux1/1
  Omega/1 -> Calc_errors/2(Omega)
  P_E/1 -> Calc_errors/3(P_E)
  Calc_errors/1(e_l) -> Gain/1, alpha_2/2(z1)  "z1"
  Add1/1 -> alpha_2/1(alpha_1), Sum/1  "alpha_1"
  Tan/1 -> Sum/2, alpha_2/4(gamma)  "gamma"
  w/1 -> Demux/1
  Demux/2 -> Terminator1/1
  Demux/1 -> Terminator/1
  Sum/1 -> Product/1, alpha_2/3(z2)  "z2"
  Demux1/3 -> Terminator2/1
  Demux1/1 -> To Workspace1/1, Divide/2, alpha_2/5(vx)  "vx"
  Demux1/2 -> Divide/1, alpha_2/6(vy)  "vy"
  Calc_errors/3(kappa_C) -> alpha_2/7(kappa_C)
  alpha_2/2(alpha_2) -> Sum1/1, Derivative/1
  Demux/3 -> Sum1/2  "r"
  Sum1/1 -> Gain2/1  "z3"
  alpha_2/1(q) -> Product/2
  Gain2/1 -> Add/2
  Derivative/1 -> Add/3
  Product/1 -> Add/1
  Add/1 -> Gain1/1
  Gain1/1 -> To Workspace/1, Tau_z/1
  Calc_errors/2(e_psi) -> Tan/1
  Gain/1 -> Add1/1  "alpha_1"
  Divide/1 -> Add1/2

== system Car_14DOF_Lat_Long_Control_FINAL/LAT_CONTROL/LSTM_NETWORK ==
  Tau_z : Inport
  rho : Inport  Port=2
  Add : Sum  Inputs=++++
  Demux : Demux
  Gain : Gain  Gain=1/4
  MATLAB Function : MATLAB Function  TreatAsAtomicUnit=on
  MATLAB Function1 : MATLAB Function  TreatAsAtomicUnit=on
  Mux : Mux  Inputs=3
  Stateful Predict : deeplib/Stateful Predict  Network=Network from MAT-file  NetworkFunction=untitled  NetworkFilePath=/media/sherlock2204/Alice/Mis_Documentos_R/Doctorado/Tesis/SimCar_MATLAB/MATLAB_F/LSTM_network.mat  InputDataFormats={'',''}  SampleTime=0.001  ForceInterpretedSim=off  EnableDLNetwork=on  LastKnownNetworkFilePath=''  LastKnownNetworkTimeStamp=''
  To Workspace : ToWorkspace  VariableName=lstm_in  SaveFormat=Timeseries  SampleTime=-1
  To Workspace1 : ToWorkspace  VariableName=rho  SaveFormat=Timeseries  SampleTime=-1
  Unit Delay : UnitDelay  SampleTime=0.001  HasFrameUpgradeWarning=on
  delta_w : Outport
  wires:
  Stateful Predict/1 -> MATLAB Function1/1(u)
  Mux/1 -> To Workspace/1, MATLAB Function/1(v)
  rho/1 -> Demux/1
  Tau_z/1 -> Mux/1
  Unit Delay/1 -> Mux/3
  Demux/4 -> Add/4
  Demux/1 -> Add/1
  Demux/2 -> Add/2
  Demux/3 -> Add/3
  Add/1 -> Gain/1
  Gain/1 -> To Workspace1/1, Mux/2
  MATLAB Function1/1(y) -> delta_w/1, Unit Delay/1
  MATLAB Function/1(y) -> Stateful Predict/1

== system Car_14DOF_Lat_Long_Control_FINAL/LONG_CONTROL/ADRC ==
  x1 : Inport
  x1_ref : Inport  Port=2
  hat_x2 : Inport  Port=3
  Add : Sum  Inputs=+++-
  Add1 : Sum  Inputs=++++
  Demux : Demux
  Derivative : Derivative
  Gain : Gain  Gain=kp
  Gain1 : Gain  Gain=ki
  Gain2 : Gain  Gain=[1;1;1;1]/reff
  Gain3 : Gain  Gain=1/4
  Integrator : Integrator
  Sum : Sum  Inputs=|+-
  To Workspace : ToWorkspace  VariableName=e_c  SaveFormat=Timeseries  SampleTime=-1
  u : Outport
  wires:
  x1/1 -> Sum/2  "rho"
  Sum/1 -> Demux/1, Gain/1, Integrator/1  "e_c"
  Integrator/1 -> Gain1/1
  Gain/1 -> Add/2
  Gain1/1 -> Add/3
  hat_x2/1 -> Add/4
  Add/1 -> u/1
  Gain2/1 -> Derivative/1, Sum/1  "rho_ref"
  Derivative/1 -> Add/1
  x1_ref/1 -> Gain2/1
  Demux/1 -> Add1/1
  Demux/3 -> Add1/3
  Demux/4 -> Add1/4
  Demux/2 -> Add1/2
  Add1/1 -> Gain3/1
  Gain3/1 -> To Workspace/1

== system Car_14DOF_Lat_Long_Control_FINAL/LONG_CONTROL/ESO ==
  x1 : Inport
  u : Inport  Port=2
  Add : Sum  Inputs=+++
  Add1 : Sum  Inputs=++++
  Demux : Demux
  Gain : Gain  Gain=L1
  Gain1 : Gain  Gain=L2
  Gain3 : Gain  Gain=1/4
  Integrator : Integrator
  Integrator1 : Integrator
  Sum : Sum  Inputs=|+-
  To Workspace : ToWorkspace  VariableName=e_o  SaveFormat=Timeseries  SampleTime=-1
  hat_x2 : Outport
  wires:
  Sum/1 -> Demux/1, Gain1/1, Gain/1  "e_o"
  Gain/1 -> Add/2
  Add/1 -> Integrator/1  "D_hat_x1"
  x1/1 -> Sum/1
  Integrator/1 -> Sum/2  "hat_x1"
  Gain1/1 -> Integrator1/1  "D_hat_x2"
  Integrator1/1 -> hat_x2/1, Add/1  "hat_x2"
  u/1 -> Add/3
  Add1/1 -> Gain3/1
  Demux/3 -> Add1/3
  Demux/2 -> Add1/2
  Demux/1 -> Add1/1
  Demux/4 -> Add1/4
  Gain3/1 -> To Workspace/1

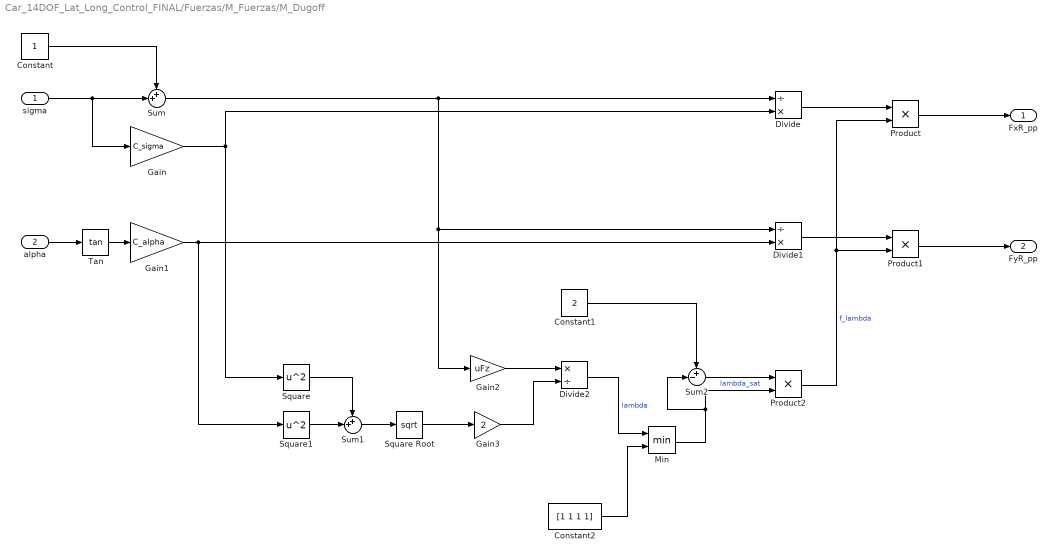
== system Car_14DOF_Lat_Long_Control_FINAL/Fuerzas/M_Fuerzas/M_Dugoff ==
  sigma : Inport
  alpha : Inport  Port=2
  Constant : Constant
  Constant1 : Constant  Value=2
  Constant2 : Constant  Value=[1 1 1 1]
  Divide : Product  Inputs=/*
  Divide1 : Product  Inputs=/*
  Divide2 : Product  Inputs=*/
  Gain : Gain  Gain=C_sigma
  Gain1 : Gain  Gain=C_alpha
  Gain2 : Gain  Gain=uFz
  Gain3 : Gain  Gain=2
  Min : MinMax  Inputs=2
  Product : Product
  Product1 : Product
  Product2 : Product
  Square : Math  Operator=square
  Square Root : Sqrt
  Square1 : Math  Operator=square
  Sum : Sum  Inputs=++|
  Sum1 : Sum  Inputs=++|
  Sum2 : Sum  Inputs=+-|
  Tan : Trigonometry  Operator=tan
  FxR_pp : Outport
  FyR_pp : Outport  Port=2
  wires:
  alpha/1 -> Tan/1
  sigma/1 -> Gain/1, Sum/2
  Constant/1 -> Sum/1
  Sum/1 -> Divide/1, Divide1/1, Gain2/1
  Gain/1 -> Square/1, Divide/2
  Divide/1 -> Product/1
  Tan/1 -> Gain1/1
  Gain1/1 -> Divide1/2, Square1/1
  Divide1/1 -> Product1/1
  Product/1 -> FxR_pp/1
  Product1/1 -> FyR_pp/1
  Gain2/1 -> Divide2/1
  Square1/1 -> Sum1/2
  Square/1 -> Sum1/1
  Sum1/1 -> Square Root/1
  Gain3/1 -> Divide2/2
  Square Root/1 -> Gain3/1
  Divide2/1 -> Min/1  "lambda"
  Constant1/1 -> Sum2/1
  Sum2/1 -> Product2/1
  Product2/1 -> Product1/2, Product/2  "f_lambda"
  Min/1 -> Product2/2, Sum2/2  "lambda_sat"
  Constant2/1 -> Min/2

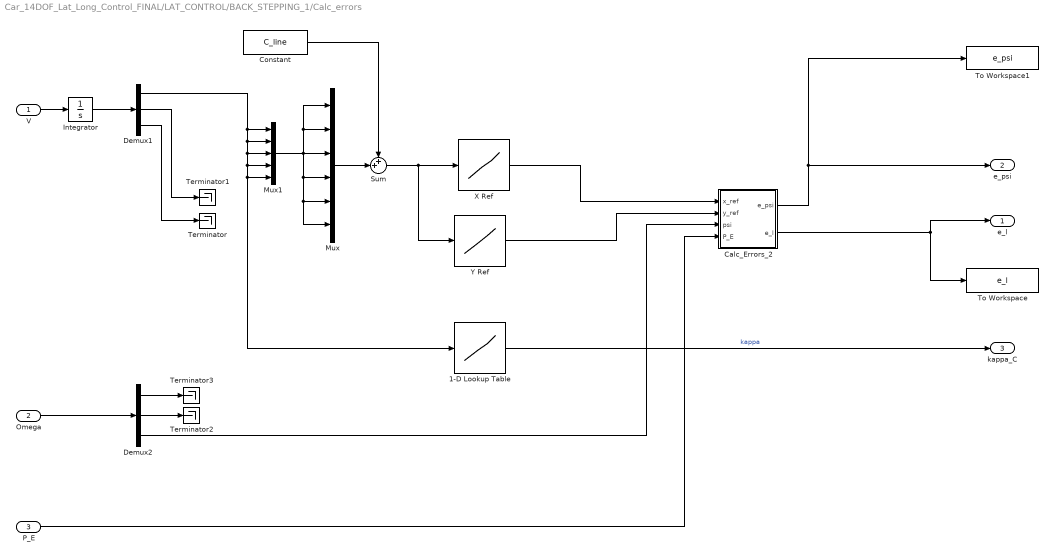
== system Car_14DOF_Lat_Long_Control_FINAL/LAT_CONTROL/BACK_STEPPING_1/Calc_errors ==
  V : Inport
  Omega : Inport  Port=2
  P_E : Inport  Port=3
  1-D Lookup Table : Lookup_n-D  NumberOfTableDimensions=1  BreakpointsForDimension1=gradbp  Table=curvature  InternalRulePriority=Speed  RndMeth=Simplest
  Calc_Errors_2 : MATLAB Function  TreatAsAtomicUnit=on
  Constant : Constant  Value=C_line
  Demux1 : Demux  Outputs=3
  Demux2 : Demux  Outputs=3
  Integrator : Integrator
  Mux : Mux  Inputs=6
  Mux1 : Mux  Inputs=5
  Sum : Sum  Inputs=++|
  Terminator{,1..3} (4 alike) : Terminator
  To Workspace : ToWorkspace  VariableName=e_l  SaveFormat=Timeseries  SampleTime=-1
  To Workspace1 : ToWorkspace  VariableName=e_psi  SaveFormat=Timeseries  SampleTime=-1
  X Ref : Lookup_n-D  NumberOfTableDimensions=1  BreakpointsForDimension1=gradbp  Table=xRef2s  InternalRulePriority=Speed  RndMeth=Simplest
  Y Ref : Lookup_n-D  NumberOfTableDimensions=1  BreakpointsForDimension1=gradbp  Table=yRef2s  InternalRulePriority=Speed  RndMeth=Simplest
  e_l : Outport
  e_psi : Outport  Port=2
  kappa_C : Outport  Port=3
  wires:
  Mux/1 -> Sum/2
  Sum/1 -> X Ref/1, Y Ref/1
  V/1 -> Integrator/1
  Demux1/1 -> 1-D Lookup Table/1, Mux1/5, Mux1/4, Mux1/3, Mux1/2, Mux1/1
  Integrator/1 -> Demux1/1
  Demux1/3 -> Terminator/1
  Constant/1 -> Sum/1
  X Ref/1 -> Calc_Errors_2/1(x_ref)
  Demux2/1 -> Terminator3/1
  Demux2/2 -> Terminator2/1
  Demux1/2 -> Terminator1/1
  Y Ref/1 -> Calc_Errors_2/2(y_ref)
  Omega/1 -> Demux2/1
  Demux2/3 -> Calc_Errors_2/3(psi)
  P_E/1 -> Calc_Errors_2/4(P_E)
  1-D Lookup Table/1 -> kappa_C/1  "kappa"
  Mux1/1 -> Mux/6, Mux/5, Mux/4, Mux/3, Mux/1, Mux/2
  Calc_Errors_2/2(e_l) -> e_l/1, To Workspace/1
  Calc_Errors_2/1(e_psi) -> To Workspace1/1, e_psi/1

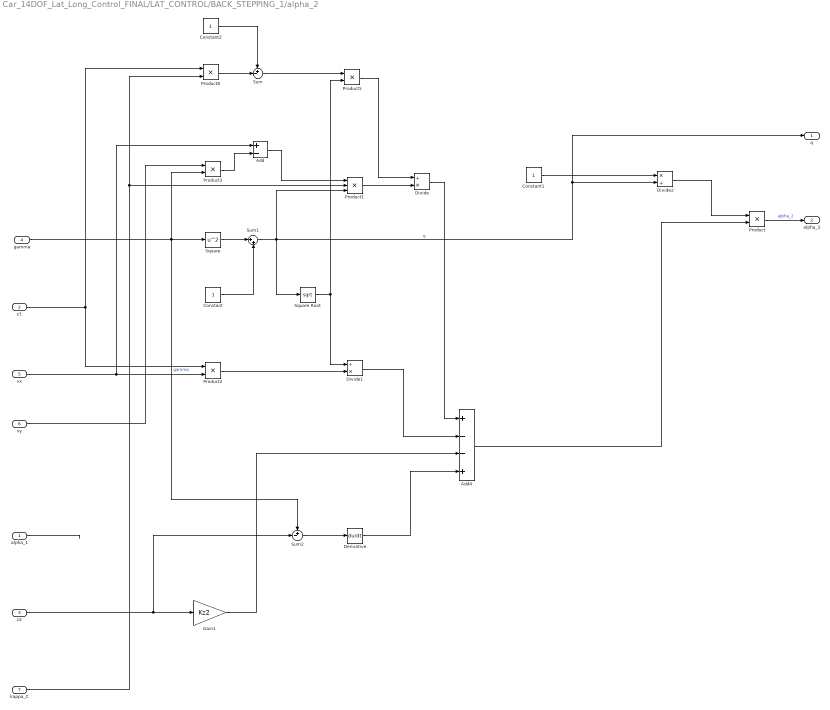
== system Car_14DOF_Lat_Long_Control_FINAL/LAT_CONTROL/BACK_STEPPING_1/alpha_2 ==
  alpha_1 : Inport
  z1 : Inport  Port=2
  z2 : Inport  Port=3
  gamma : Inport  Port=4
  vx : Inport  Port=5
  vy : Inport  Port=6
  kappa_C : Inport  Port=7
  Add : Sum  Inputs=+-
  Add4 : Sum  Inputs=+--+
  Constant : Constant
  Constant1 : Constant
  Constant2 : Constant
  Derivative : Derivative
  Divide : Product  Inputs=/*
  Divide1 : Product  Inputs=/*
  Divide2 : Product  Inputs=*/
  Gain1 : Gain  Gain=Kz2
  Product{,2..3,5,8} (5 alike) : Product
  Product1 : Product  Inputs=3
  Square : Math  Operator=square
  Square Root : Sqrt
  Sum : Sum  Inputs=+-|
  Sum1 : Sum  Inputs=|++
  Sum2 : Sum  Inputs=+-|
  q : Outport
  alpha_2 : Outport  Port=2
  wires:
  Constant/1 -> Sum1/2
  Square/1 -> Sum1/1
  gamma/1 -> Square/1, Sum2/1, Product3/2  "gamma"
  Sum1/1 -> Divide2/2, q/1, Product1/3, Square Root/1  "q"
  vx/1 -> Add/1, Product2/2
  z1/1 -> Product8/1, Product2/1
  vy/1 -> Product3/1
  z2/1 -> Gain1/1, Sum2/2
  kappa_C/1 -> Product1/2, Product8/2
  Gain1/1 -> Add4/3
  Product2/1 -> Divide1/2
  Add/1 -> Product1/1
  Product3/1 -> Add/2
  Product1/1 -> Divide/2
  Constant2/1 -> Sum/1
  Product8/1 -> Sum/2
  Add4/1 -> Product/2
  Product/1 -> alpha_2/1  "alpha_2"
  Sum/1 -> Product5/1
  Square Root/1 -> Divide1/1, Product5/2
  Product5/1 -> Divide/1
  Divide/1 -> Add4/1
  Divide1/1 -> Add4/2
  Derivative/1 -> Add4/4
  alpha_1/1 -> ?
  Divide2/1 -> Product/1
  Constant1/1 -> Divide2/1
  Sum2/1 -> Derivative/1

== matlab function Car_14DOF_Lat_Long_Control_FINAL/LAT_CONTROL/LSTM_NETWORK/MATLAB Function1 ==
  data: u input; y output
function y = fcn(u)

y = 0.7854*double(u);

== matlab function Car_14DOF_Lat_Long_Control_FINAL/LAT_CONTROL/LSTM_NETWORK/MATLAB Function ==
  data: v input; y output
function y = fcn(v)
% if isnan(v(1))==1
%     v(1) = 0;
% end

tau_z = (1/13641.0)*v(1);
rho = (1/150.0)*v(2);
dw = (1/0.7854)*v(3);
y = [tau_z; rho; dw];

== matlab function Car_14DOF_Lat_Long_Control_FINAL/LAT_CONTROL/BACK_STEPPING_1/Calc_errors/Calc_Errors_2 ==
  data: x_ref input; e_psi output; y_ref input; psi input; P_E input; e_l output
function [e_psi, e_l] = fcn(x_ref,y_ref,psi,P_E)

P = polyfit(x_ref,y_ref,1);
m2 = P(1);
b2 = P(2);
x1 = 0;
y1 = b2;
x2 = 1;
y2 = m2*x2+b2;
psi_ref = atan2(y2-y1,x2-x1);
%psi_ref = atan(m);
e_psi = psi-psi_ref;

% Traslacion al lugar donde esta el punto S
x_s = P_E(1)-x_ref(16);
y_s = P_E(2)-y_ref(16);
% Rotacion a la misma orientacion del coche
y_c = x_s*sin(-psi_ref)+y_s*cos(-psi_ref);
e_l = y_c;
